simulink model "string_perhaps"  (R2020a)
settings: Solver=VariableStepAuto  StartTime=0.0  StopTime=10  RelTol=1e-3
values from neighbouring files (symbols this model uses):
  a = [1 zeros(1, delay) -0.5 -0.5]    [callidk.m]
  b = firls(42, [0 1/delay 2/delay 1], [0 0 1 1])    [callidk.m]
  delay = round(Fs/A)    [callidk.m]    (also in sons.m = round(Fs/f); sons2.m = round(Fs/f); sons3.m = round(Fs/f))
  g0 = g_cte*(1+B)/2    [callidk.m]
  g1 = g_cte*(1-B)/4    [callidk.m]
  Ts = 1/Fs    (= 2.27272727273e-05)    [callidk.m]    (also in sons.m = 2.26757369615e-05; sons2.m = 2.26757369615e-05; sons3.m = 2.26757369615e-05)
libraries: simulink x3, cstblocks x1
settings Model: Creator=Jose Murteira  LastModifiedBy=Jose Murteira

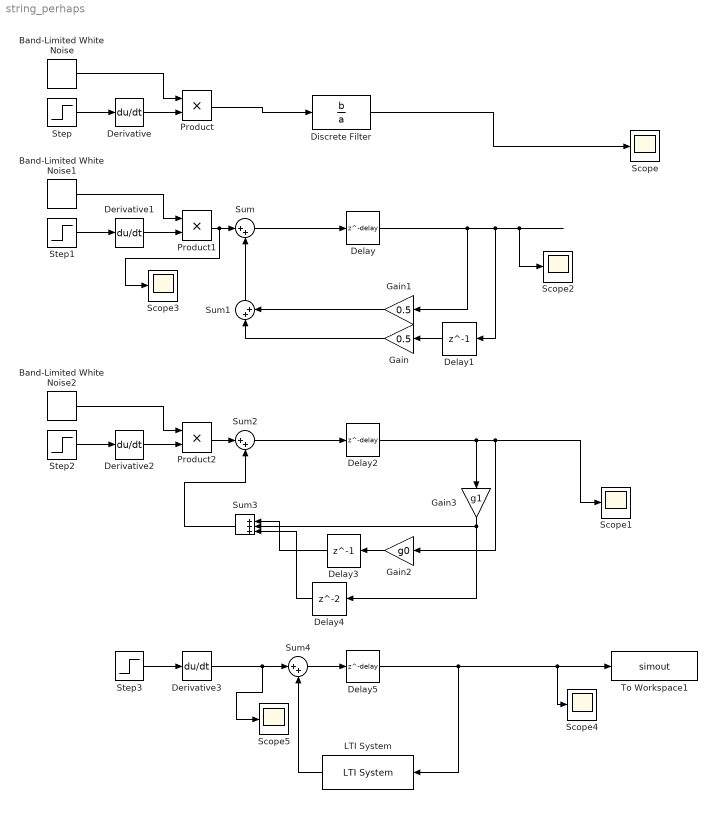
== system string_perhaps ==
  Band-Limited White Noise : simulink/Sources/Band-Limited White Noise  Cov=[0.01]  Ts=Ts  seed=[23341]
  Band-Limited White Noise1 : simulink/Sources/Band-Limited White Noise  Cov=[0.01]  Ts=Ts  seed=[23341]
  Band-Limited White Noise2 : simulink/Sources/Band-Limited White Noise  Cov=[0.01]  Ts=Ts  seed=[23341]
  Delay : Delay  DelayLength=delay  InitialCondition=0  SampleTime=Ts
  Delay1 : Delay  DelayLength=1  InitialCondition=0
  Delay2 : Delay  DelayLength=delay  InitialCondition=0  SampleTime=Ts
  Delay3 : Delay  DelayLength=1  InitialCondition=0
  Delay4 : Delay  InitialCondition=0
  Delay5 : Delay  DelayLength=delay  InitialCondition=0  SampleTime=Ts
  Derivative{,1..3} (4 alike) : Derivative
  Discrete Filter : DiscreteFilter  Numerator=b  Denominator=a  SampleTime=Ts
  Gain : Gain  Gain=0.5
  Gain1 : Gain  Gain=0.5
  Gain2 : Gain  Gain=g0
  Gain3 : Gain  Gain=g1
  LTI System : cstblocks/LTI System  sys=le_tf  IC=[]
  Product : Product
  Product1 : Product
  Product2 : Product
  Scope{,1..5} (6 alike) : Scope
  Step{,1..3} (4 alike) : Step  Time=0.01  SampleTime=1/44000
  Sum{,1..2,4} (4 alike) : Sum  Inputs=|++
  Sum3 : Sum  Inputs=|+++
  To Workspace1 : ToWorkspace  VariableName=simout  SaveFormat=Timeseries  SampleTime=-1
  wires:
  Step/1 -> Derivative/1
  Derivative/1 -> Product/2
  Band-Limited White Noise/1 -> Product/1
  Product/1 -> Discrete Filter/1
  Step1/1 -> Derivative1/1
  Band-Limited White Noise1/1 -> Product1/1
  Derivative1/1 -> Product1/2
  Product1/1 -> Scope3/1, Sum/1
  Sum/1 -> Delay/1
  Discrete Filter/1 -> Scope/1
  Delay/1 -> Gain1/1, Delay1/1, Scope2/1
  Delay1/1 -> Gain/1
  Gain1/1 -> Sum1/2
  Gain/1 -> Sum1/1
  Sum1/1 -> Sum/2
  Step2/1 -> Derivative2/1
  Gain3/1 -> Delay4/1, Sum3/2
  Derivative2/1 -> Product2/2
  Gain2/1 -> Delay3/1
  Product2/1 -> Sum2/1
  Sum3/1 -> Sum2/2
  Band-Limited White Noise2/1 -> Product2/1
  Sum2/1 -> Delay2/1
  Delay3/1 -> Sum3/1
  Delay2/1 -> Gain2/1, Scope1/1, Gain3/1
  Delay4/1 -> Sum3/3
  Sum4/1 -> Delay5/1
  LTI System/1 -> Sum4/2
  Derivative3/1 -> Scope5/1, Sum4/1
  Step3/1 -> Derivative3/1
  Delay5/1 -> To Workspace1/1, Scope4/1, LTI System/1
